simulink model "full_controlled"  (R2023a)
settings: Solver=VariableStepAuto  StartTime=0.0  StopTime=0.5  RelTol=1e-3
undefined symbols (not defined in the file): a
libraries: spsThyristorLib x4, spsACVoltageSourceLib x1, spsDCMachineLib x1, spsDCVoltageSourceLib x1, spsVoltageMeasurementLib x1, sps_lib x1
settings Model: Creator=Arnesh S  LastModifiedBy=Arnesh S

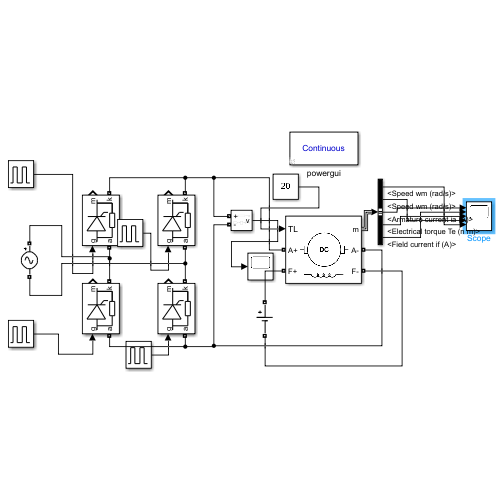
[thumbnail: Simulink's stored preview of the top-level diagram]
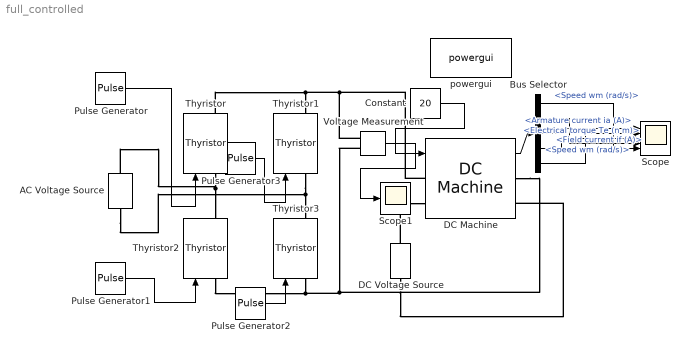
== system full_controlled ==
  AC Voltage Source : spsACVoltageSourceLib/AC Voltage Source  Amplitude=320  Phase=0  Frequency=50  SampleTime=0  Measurements=None  BusType=swing  Pref=10e3  Qref=0  Qmin=-inf  Qmax=+inf
  Bus Selector : BusSelector  OutputSignals=Speed wm (rad/s),Speed wm (rad/s),Armature current ia (A),Electrical torque Te (n m),Field current if (A)
  Constant : Constant  Value=20
  DC Machine : spsDCMachineLib/DC Machine  PresetModel=01: 5HP 240V 1750RPM Field:300V  MechanicalLoad=Torque TL  FieldType=Wound  ShowDetailedParameters=on  MeasurementBus=off  RLa=[2.581 0.028]  RLf=[281.2 156]  Laf=0.9483  MachineConstant=Torque constant (N.m/A)  Ke=1.8  Kt=1.8  J=0.02215  Bm=0.002953  Tf=0.5161  w0=1  Ifinit=1.06685632871799  TsPowergui=0  TsBlock=-1
  DC Voltage Source : spsDCVoltageSourceLib/DC Voltage Source  Amplitude=300  Measurements=None
  Pulse Generator : DiscretePulseGenerator  PulseType=Time based  Period=1/50  PulseWidth=5  PhaseDelay=(a*0.02)/360
  Pulse Generator1 : DiscretePulseGenerator  PulseType=Time based  Period=1/50  PulseWidth=5  PhaseDelay=(a+180)*0.02/360
  Pulse Generator2 : DiscretePulseGenerator  PulseType=Time based  Period=1/50  PulseWidth=5  PhaseDelay=(a*0.02)/360
  Pulse Generator3 : DiscretePulseGenerator  PulseType=Time based  Period=1/50  PulseWidth=5  PhaseDelay=(a+180)*0.02/360
  Scope : Scope  NumInputPorts=5
  Scope1 : Scope
  Thyristor{,1..3} (4 alike) : spsThyristorLib/Thyristor  Ron=0.001  Lon=0  Vf=0.8  IC=0  Rs=500  Cs=250e-9  Measurements=on
  Voltage Measurement : spsVoltageMeasurementLib/Voltage Measurement  PhasorSimulation=off  OutputType=Complex  PSBequivalent=0
  powergui : sps_lib/powergui  Priority=1  SimulationMode=Continuous  SampleTime=50e-6  frequency=60  Iterations=50  frequencyindice=0  Pbase=100e6  ErrMax=1e-4  UnitsV=kV  UnitsW=MW  buscounter=0  FunctionMessages=off  echomessages=off  EnableUseOfTLC=off  CurrentSourceSwitches=off  DisableSnubberDevices=off  DisableRonSwitches=off  DisableVfSwitches=off  DisplayEquations=off  AutomaticDiscreteSolvers=off  SolverType=Tustin/Backward Euler (TBE)  Interpol=off  ExternalGateDelay=off  methode=off  Ts=100  x0status=blocks  SPID=on  SwTol=0  HookPort=off  NonlinearTolerance=1e-4  nMaxIteration=100  ContinueOnMaxIteration=off  RestoreLinks=warning  ResistiveCurrentMeasurement=off  Frange=[0:2:500]  Ylog=off  Xlog=on  ShowGrid=off  save=off  variable=ZData  structure=0  ZoomFFT=off  StartTime=0.0  cycles=1  DisplayStyle=1  fundamental=60  FreqAxis=off  MaxFrequency=1000  frequencyindicesteady=1  RmsSteady=1  display=off
  wires:
  Pulse Generator/1 -> Thyristor/1
  Pulse Generator1/1 -> Thyristor2/1
  Pulse Generator3/1 -> Thyristor1/1
  Pulse Generator2/1 -> Thyristor3/1
  Constant/1 -> DC Machine/1
  DC Machine/1 -> Bus Selector/1
  Bus Selector/1 -> Scope/5  "<Speed wm (rad/s)>"
  Bus Selector/2 -> Scope/4  "<Speed wm (rad/s)>"
  Bus Selector/3 -> Scope/1  "<Armature current ia (A)>"
  Bus Selector/4 -> Scope/3  "<Electrical torque Te (n m)>"
  Bus Selector/5 -> Scope/2  "<Field current if (A)>"
  Voltage Measurement/1 -> Scope1/1
  connections:
  AC Voltage Source/LConn1 -- Thyristor1/LConn1 -- Thyristor3/RConn1
  AC Voltage Source/RConn1 -- Thyristor/LConn1 -- Thyristor2/RConn1
  Voltage Measurement/LConn2 -- DC Machine/RConn1 -- Thyristor2/LConn1 -- Thyristor3/LConn1
  Voltage Measurement/LConn1 -- DC Machine/LConn1 -- Thyristor/RConn1 -- Thyristor1/RConn1
  DC Voltage Source/RConn1 -- DC Machine/LConn2
  DC Voltage Source/LConn1 -- DC Machine/RConn2
